simulink model "RefModel_SimpleUavMotion"  (R2020a)
settings: Solver=ode1  StartTime=0.0  StopTime=10.0  FixedStep=Ts_Task.Ts_base  RelTol=1e-3
undefined symbols (not defined in the file or in its folder): alt, DiscIntNeverNeededParam, ENUM_FlightControlMode, ENUM_UAVMode, eulerd_yaw_pitch_roll, initialAlignmentCompleteFlag, isHeadingRotateFlag, isNavFilterGood, latd, lla, lond, pitchd, posNED, refloc, rolld, TASK_SET, Ts_SimpleUavMotion, velNED, yawd
libraries: simulink x16, discretizedSecondOrderIntegrator x3, discretizing x2
(part 1 of 2)
settings Model: Creator=sl  LastModifiedBy=Administrator
settings DataIOCC: SaveOutput=off  SaveTime=off
settings OptimizationCC: DefaultParameterBehavior=Inlined  EnhancedBackFolding=on  PassReuseOutputArgsAs=Individual arguments  ZeroExternalMemoryAtStartup=off  ZeroInternalMemoryAtStartup=off  OptimizeBlockOrder=speed  DifferentSizesBufferReuse=on  EfficientTunableParamExpr=on
settings DebuggingCC: InheritedTsInSrcMsg=none  ParameterPrecisionLossMsg=none  ParameterTunabilityLossMsg=error  UnconnectedInputMsg=none  UnconnectedOutputMsg=none  UnconnectedLineMsg=none  SFUnusedDataAndEventsDiag=none
settings HardwareCC: ProdBitPerPointer=32  ProdBitPerSizeT=32  ProdBitPerPtrDiffT=32  ProdLargestAtomicInteger=Long  ProdLargestAtomicFloat=Double  ProdWordSize=32  ProdHWDeviceType=ARM Compatible->ARM Cortex
settings ModelReferenceCC: ModelReferenceNumInstancesAllowed=Single
settings SFSimCC: MATLABDynamicMemAlloc=off
settings RTWCC: SystemTargetFile=ert.tlc  TemplateMakefile=ert_default_tmf  GenerateReport=on  IncludeHyperlinkInReport=on  LaunchReport=on  GenerateTraceInfo=on  GenerateTraceReport=on  GenerateTraceReportSl=on  GenerateTraceReportSf=on  GenerateTraceReportEml=on
settings CodeAppCC: ForceParamTrailComments=on  IgnoreCustomStorageClasses=off  MaxIdLength=48  OperatorAnnotations=on  SimulinkDataObjDesc=on  SFDataObjDesc=on  InsertBlockDesc=on
settings ERTTargetCC: TargetLangStandard=C99 (ISO)  GenerateSampleERTMain=on  CombineOutputUpdateFcns=off  LogVarNameModifier=none  SupportVariableSizeSignals=on  InlinedParameterPlacement=NonHierarchical  ERTCustomFileTemplate=example_file_process.tlc

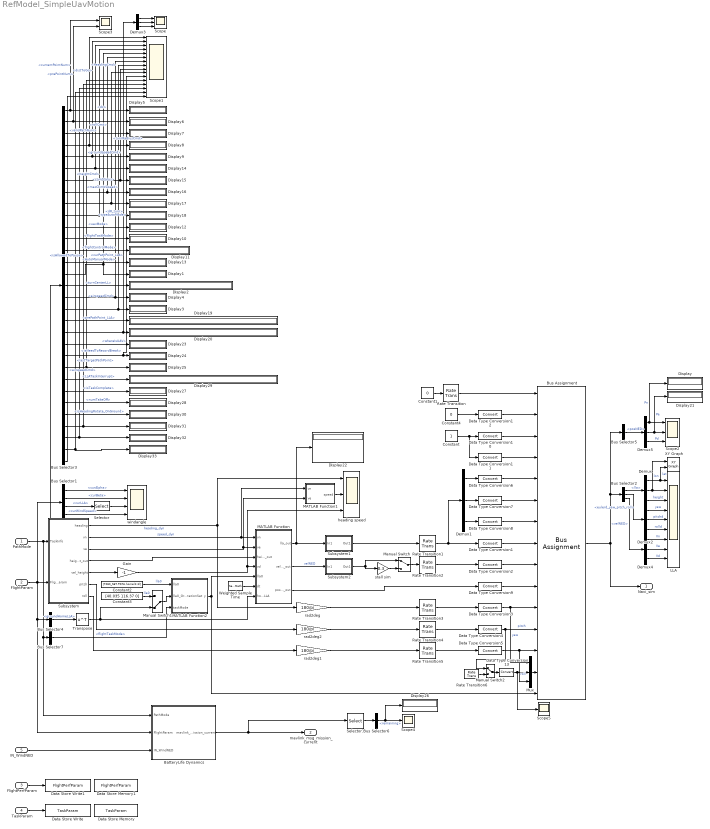
== system RefModel_SimpleUavMotion ==
  PathMode : Inport  OutDataTypeStr=Bus: BUS_TASK_PATH_OutParam
  FlightParam : Inport  Port=2  OutDataTypeStr=Bus: BUS_TASK_COMMON_OutParam
  FlightPerfParam : Inport  Port=3  OutDataTypeStr=Bus: BUS_FLIGHTPERF_PARAM  BusOutputAsStruct=on
  TaskParam : Inport  Port=4  OutDataTypeStr=Bus: BUS_TASK_PATH_AlgoParam  BusOutputAsStruct=on
  IN_WindNED : Inport  Port=5  OutDataTypeStr=Bus: BUS_NAVI_GlobalWindEst
  BatteryLife Dynamics : Subsystem
  Bus Assignment : BusAssignment  AssignedSignals=isHeadingRotateFlag,initialAlignmentCompleteFlag,isNavFilterGood,latd,lond,alt,lla,velNED,posNED,yawd,pitchd,rolld,eulerd_yaw_pitch_roll,refloc
  Bus Selector1 : BusSelector  OutputSignals=curAlpha,curBeta,curLLA,curWindSpeed
  Bus Selector2 : BusSelector  OutputSignals=lla,eulerd_yaw_pitch_roll,velNED
  Bus Selector3 : BusSelector  OutputSignals=currentPointNum,prePointNum,validPathNum,headingCmd,distToGo,dz,groundspeedCmd,rollCmd,turnRadiusCmd,heightCmd,uavMode,flightTaskMode,flightControlMode,AutoManualMode,dR_turn,turnCenterLL,comStatus,maxClimbSpeed,prePathPoint_LLA,curPathPoint_LLA,whereIsUAV,typeAutoMode,airspeedCmd,LLATaskInterrupt,isTaskComplete,numTakeOff,isHeadingRotate_OnGround,isAllowedToPause,isNeedToRecordBreak,lastTargetPathPoint,airspeedCmd
  Bus Selector4 : BusSelector  OutputSignals=groundHomeLLA
  Bus Selector5 : BusSelector  OutputSignals=posNED
  Bus Selector6 : BusSelector  OutputSignals=remaining
  Bus Selector7 : BusSelector  OutputSignals=flightTaskMode
  Constant : Constant
  Constant1 : Constant  Value=0  OutDataTypeStr=Bus: BUS_NAVI_TO_FIRM
  Constant2 : Constant  Value=[TASK_SET.PATH.home(1:3)]
  Constant3 : Constant  Value=[40.035 116.37 0]
  Constant4 : Constant  Value=0
  Data Store Memory : DataStoreMemory  DataStoreName=TaskParam  ReadBeforeWriteMsg=warning  WriteAfterWriteMsg=warning  WriteAfterReadMsg=warning  ShowAdditionalParam=off  OutDataTypeStr=Bus: BUS_TASK_PATH_AlgoParam  Dimensions=1
  Data Store Memory1 : DataStoreMemory  DataStoreName=FlightPerfParam  ReadBeforeWriteMsg=warning  WriteAfterWriteMsg=warning  WriteAfterReadMsg=warning  ShowAdditionalParam=off  OutDataTypeStr=Bus: BUS_FLIGHTPERF_PARAM  Dimensions=1
  Data Store Write : DataStoreWrite  DataStoreName=TaskParam
  Data Store Write1 : DataStoreWrite  DataStoreName=FlightPerfParam
  Data Type Conversion{1..13} (13 alike) : DataTypeConversion
  Demux{,1..5} (6 alike) : Demux  Outputs=3
  Display{,1..33} (34 alike) : Display
  Gain : Gain  Gain=-1
  LLA : Scope  NumInputPorts=9
  MATLAB Function : MATLAB Function  TreatAsAtomicUnit=on
  MATLAB Function1 : MATLAB Function  TreatAsAtomicUnit=on
  MATLAB Function2 : MATLAB Function  TreatAsAtomicUnit=on
  Manual Switch : ManualSwitch
  Manual Switch1 : ManualSwitch  CurrentSetting=0
  Manual Switch2 : ManualSwitch
  Mux : Mux  Inputs=3
  Rate Transition{,1..6} (7 alike) : RateTransition
  Scope : Scope  NumInputPorts=3
  Scope1 : Scope  NumInputPorts=16
  Scope2 : Scope  NumInputPorts=3
  Scope3 : Scope  NumInputPorts=2
  Scope4 : Scope
  Scope5 : Scope
  Selector : Selector  InputPortWidth=3  IndexOptions=Index vector (dialog)  Indices=3  OutputSizes=1
  Selector1 : Selector  InputPortWidth=3  IndexOptions=Index vector (dialog)  Indices=1  OutputSizes=1
  Subsystem : Subsystem
  Subsystem1 : Subsystem
  Subsystem2 : Subsystem
  Transpose : Math  Operator=transpose  SaturateOnIntegerOverflow=on
  Weighted Sample Time : SampleTimeMath  TsampMathOp=Ts Only
  XY Graph : simulink/Sinks/XY Graph  xmin=116.34  xmax=116.42  ymin=40.02  ymax=40.08  st=-1
  heading speed : Scope  NumInputPorts=3
  rad2deg : Gain  Gain=180/pi
  rad2deg1 : Gain  Gain=180/pi
  rad2deg2 : Gain  Gain=180/pi
  stall sim : Gain  Gain=0.3
  windangle : Scope  NumInputPorts=4
  Navi_sim : Outport  OutDataTypeStr=Bus: BUS_NAVI_TO_FIRM
  mavlink_msg_mission_current : Outport  Port=2  OutDataTypeStr=Bus: mavlink_msg_mission_current  BusOutputAsStruct=on
  wires:
  Data Type Conversion2/1 -> Bus Assignment/9
  Bus Selector3/16 -> Display2/1  "<turnCenterLL>"
  Rate Transition5/1 -> Data Type Conversion5/1
  Data Type Conversion5/1 -> Mux/3, Bus Assignment/13  "roll"
  Bus Selector3/15 -> Display1/1, Scope1/5  "<dR_turn>"
  Weighted Sample Time/1 -> MATLAB Function/6(dt)
  Data Type Conversion4/1 -> Manual Switch2/1, Bus Assignment/12  "pitch"
  Data Type Conversion1/1 -> Bus Assignment/8
  Rate Transition4/1 -> Data Type Conversion4/1
  Bus Selector3/14 -> Display13/1  "<AutoManualMode>"
  Subsystem/4(height_out) -> MATLAB Function/3(height_out)
  Data Type Conversion7/1 -> Bus Assignment/6
  Data Type Conversion6/1 -> Bus Assignment/5
  Subsystem/6(pitch) -> rad2deg2/1
  Demux1/3 -> Data Type Conversion8/1
  Rate Transition1/1 -> Demux1/1, Data Type Conversion1/1
  Data Type Conversion8/1 -> Bus Assignment/7
  Demux1/2 -> Data Type Conversion7/1
  Demux1/1 -> Data Type Conversion6/1
  Bus Selector3/13 -> Display11/1  "<flightControlMode>"
  Bus Selector3/6 -> Scope1/3, Display14/1  "<dz>"
  rad2deg1/1 -> Rate Transition5/1
  Rate Transition/1 -> Bus Assignment/1
  PathMode/1 -> Bus Selector7/1, BatteryLife Dynamics/1(PathMode), Bus Selector3/1, Subsystem/1(TaskInfo)
  Bus Selector3/2 -> Scope3/2, Display6/1  "<prePointNum>"
  Bus Selector3/8 -> Scope1/6, Display16/1  "<rollCmd>"
  Bus Selector3/10 -> Scope1/4, Display18/1  "<heightCmd>"
  Bus Selector3/1 -> Scope3/1, Display5/1  "<currentPointNum>"
  Bus Selector3/7 -> Scope1/9, Display15/1  "<groundspeedCmd>"
  Bus Selector3/5 -> Scope1/2, Display9/1  "<distToGo>"
  Constant2/1 -> MATLAB Function2/1(lla0)  "lla0"
  Bus Selector3/4 -> Scope1/1, Display8/1  "<headingCmd>"
  rad2deg/1 -> Rate Transition3/1
  Bus Selector3/11 -> Display12/1  "<uavMode>"
  Subsystem/2(vn) -> MATLAB Function1/1(vn), MATLAB Function/1(vn)  "speed_dyn"
  Subsystem/1(heading) -> heading speed/1, rad2deg/1  "heading_dyn"
  Bus Selector3/9 -> Scope1/10, Display17/1  "<turnRadiusCmd>"
  Rate Transition2/1 -> Data Type Conversion2/1
  Bus Selector3/3 -> Display7/1  "<validPathNum>"
  Bus Selector3/12 -> Display10/1  "<flightTaskMode>"
  Subsystem/5(vel_height) -> Gain/1
  Constant1/1 -> Rate Transition/1
  Subsystem/7(roll) -> rad2deg1/1
  Data Type Conversion3/1 -> Mux/1, Bus Assignment/11  "yaw"
  Mux/1 -> Bus Assignment/14
  FlightParam/1 -> BatteryLife Dynamics/2(FlightParam), Bus Selector4/1, Bus Selector1/1, Subsystem/2(FlightParam)
  rad2deg2/1 -> Rate Transition4/1
  Subsystem/3(ve) -> MATLAB Function1/2(ve), MATLAB Function/2(ve)
  MATLAB Function1/1(speed) -> heading speed/2
  MATLAB Function/2(velNED_out) -> Subsystem2/1(In1)  "velNED"
  Manual Switch/1 -> Rate Transition2/1
  stall sim/1 -> Manual Switch/2
  Demux2/2 -> LLA/5  "pitchd"
  Demux2/3 -> LLA/6  "rolld"
  Demux/1 -> XY Graph/2, LLA/1  "lat"
  Bus Assignment/1 -> Bus Selector2/1, Bus Selector5/1, Navi_sim/1
  Demux/3 -> LLA/3  "height"
  Demux2/1 -> LLA/4  "yaw"
  Demux/2 -> XY Graph/1, LLA/2  "lon"
  Bus Selector2/2 -> Demux2/1  "<eulerd_yaw_pitch_roll>"
  Bus Selector2/1 -> Demux/1  "<lla>"
  Bus Selector3/17 -> Scope1/7, Display4/1  "<comStatus>"
  Bus Selector3/18 -> Scope1/8, Display3/1  "<maxClimbSpeed>"
  Bus Selector3/20 -> Demux3/1, Display20/1  "<curPathPoint_LLA>"
  Rate Transition3/1 -> Data Type Conversion3/1
  Demux3/1 -> Scope/1
  Demux3/2 -> Scope/2
  Demux3/3 -> Scope/3
  MATLAB Function/1(lla_out) -> Display22/1, Subsystem1/1(In1)
  Subsystem1/1(Out1) -> Rate Transition1/1
  Subsystem2/1(Out1) -> Manual Switch/1, stall sim/1
  FlightPerfParam/1 -> Data Store Write1/1
  MATLAB Function2/1(y) -> MATLAB Function/5(lla0), Bus Assignment/15
  Manual Switch1/1 -> MATLAB Function2/2(lla0_GroundStationSet)
  Bus Selector4/1 -> Transpose/1  "<groundHomeLLA>"
  Constant3/1 -> Manual Switch1/1  "lla0"
  Bus Selector1/1 -> windangle/1  "<curAlpha>"
  Bus Selector1/2 -> windangle/2  "<curBeta>"
  Bus Selector2/3 -> Demux4/1  "<velNED>"
  Demux4/1 -> LLA/7  "Vn"
  Demux4/2 -> LLA/8  "Ve"
  Demux4/3 -> LLA/9  "Vd"
  Transpose/1 -> Manual Switch1/2, MATLAB Function/7(homeLLA)
  Bus Selector1/3 -> Selector/1  "<curLLA>"
  Selector/1 -> windangle/3
  Bus Selector1/4 -> windangle/4  "<curWindSpeed>"
  Gain/1 -> heading speed/3, MATLAB Function/4(vd)
  Data Type Conversion9/1 -> Bus Assignment/10
  Demux5/1 -> Display/1, Scope2/1  "Pn"
  Demux5/2 -> Display21/1, Scope2/2  "Pe"
  Demux5/3 -> Scope2/3  "Pd"
  Bus Selector5/1 -> Demux5/1  "<posNED>"
  MATLAB Function/3(posNED_out) -> Data Type Conversion9/1
  Constant/1 -> Data Type Conversion11/1, Data Type Conversion10/1
  Data Type Conversion10/1 -> Bus Assignment/3
  Bus Selector3/19 -> Display19/1  "<prePathPoint_LLA>"
  Bus Selector3/21 -> Display23/1  "<whereIsUAV>"
  Bus Selector3/22 -> Scope1/11, Display24/1  "<typeAutoMode>"
  Bus Selector3/23 -> Display25/1, Scope1/12  "<airspeedCmd>"
  Data Type Conversion11/1 -> Bus Assignment/4
  BatteryLife Dynamics/1(mavlink_msg_mission_current) -> Selector1/1, mavlink_msg_mission_current/1
  Selector1/1 -> Bus Selector6/1
  Bus Selector6/1 -> Display26/1, Scope4/1  "<remaining>"
  Bus Selector7/1 -> MATLAB Function2/3(taskMode)  "<flightTaskMode>"
  Bus Selector3/24 -> Display29/1  "<LLATaskInterrupt>"
  Bus Selector3/25 -> Display27/1  "<isTaskComplete>"
  Bus Selector3/26 -> Display28/1  "<numTakeOff>"
  Constant4/1 -> Data Type Conversion12/1
  Data Type Conversion12/1 -> Bus Assignment/2
  Bus Selector3/27 -> Display30/1  "<isHeadingRotate_OnGround>"
  IN_WindNED/1 -> BatteryLife Dynamics/3(IN_WindNED)
  Bus Selector3/28 -> Scope1/13, Display31/1  "<isAllowedToPause>"
  Bus Selector3/29 -> Scope1/14, Display32/1  "<isNeedToRecordBreak>"
  Bus Selector3/30 -> Display33/1, Scope1/15  "<lastTargetPathPoint>"
  Bus Selector3/31 -> Scope1/16  "<airspeedCmd>"
  TaskParam/1 -> Data Store Write/1
  ? -> Rate Transition6/1
  Manual Switch2/1 -> Data Type Conversion13/1
  Data Type Conversion13/1 -> Scope5/1, Mux/2
  Rate Transition6/1 -> Manual Switch2/2

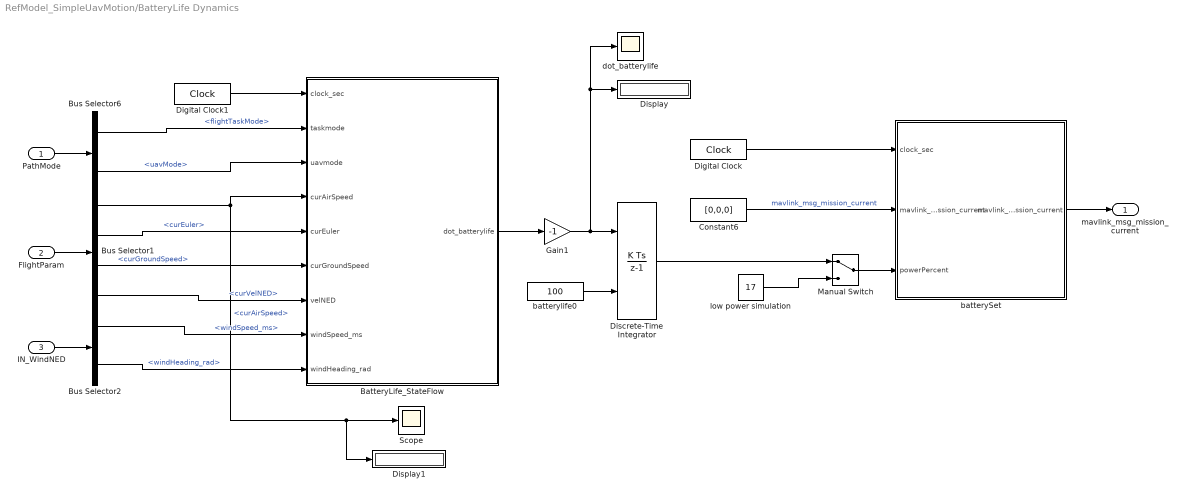
== system RefModel_SimpleUavMotion/BatteryLife Dynamics ==
  PathMode : Inport
  FlightParam : Inport  Port=2
  IN_WindNED : Inport  Port=3
  BatteryLife_StateFlow : Stateflow chart  TreatAsAtomicUnit=on
  Bus Selector1 : BusSelector  OutputSignals=curAirSpeed,curEuler,curGroundSpeed,curVelNED
  Bus Selector2 : BusSelector  OutputSignals=windSpeed_ms,windHeading_rad
  Bus Selector6 : BusSelector  OutputSignals=flightTaskMode,uavMode
  Constant6 : Constant  Value=[0,0,0]  OutDataTypeStr=Bus: mavlink_msg_mission_current
  Digital Clock : DigitalClock  SampleTime=-1
  Digital Clock1 : DigitalClock  SampleTime=-1
  Discrete-Time Integrator : DiscreteIntegrator  InitialConditionSource=external  SampleTime=-1  ICPrevOutput=DiscIntNeverNeededParam  ICPrevScaledInput=DiscIntNeverNeededParam
  Display : Display
  Display1 : Display
  Gain1 : Gain  Gain=-1
  Manual Switch : ManualSwitch
  Scope : Scope
  batterySet : MATLAB Function  TreatAsAtomicUnit=on
  batterylife0 : Constant  Value=100
  dot_batterylife : Scope
  low power simulation : Constant  Value=17
  mavlink_msg_mission_current : Outport  OutDataTypeStr=Bus: mavlink_msg_mission_current  BusOutputAsStruct=on
  wires:
  batterylife0/1 -> Discrete-Time Integrator/2
  Gain1/1 -> dot_batterylife/1, Display/1, Discrete-Time Integrator/1
  Digital Clock1/1 -> BatteryLife_StateFlow/1(clock_sec)
  BatteryLife_StateFlow/1(dot_batterylife) -> Gain1/1
  Bus Selector6/1 -> BatteryLife_StateFlow/2(taskmode)  "<flightTaskMode>"
  Constant6/1 -> batterySet/2("mavlink_msg_mission_current ")  "mavlink_msg_mission_current"
  batterySet/1(mavlink_msg_mission_current) -> mavlink_msg_mission_current/1
  Digital Clock/1 -> batterySet/1(clock_sec)
  Bus Selector6/2 -> BatteryLife_StateFlow/3(uavmode)  "<uavMode>"
  PathMode/1 -> Bus Selector6/1
  FlightParam/1 -> Bus Selector1/1
  Bus Selector1/1 -> Display1/1, Scope/1, BatteryLife_StateFlow/4(curAirSpeed)  "<curAirSpeed>"
  Bus Selector1/2 -> BatteryLife_StateFlow/5(curEuler)  "<curEuler>"
  IN_WindNED/1 -> Bus Selector2/1
  Bus Selector2/1 -> BatteryLife_StateFlow/8(windSpeed_ms)  "<windSpeed_ms>"
  Bus Selector2/2 -> BatteryLife_StateFlow/9(windHeading_rad)  "<windHeading_rad>"
  Bus Selector1/3 -> BatteryLife_StateFlow/6(curGroundSpeed)  "<curGroundSpeed>"
  Discrete-Time Integrator/1 -> Manual Switch/1
  low power simulation/1 -> Manual Switch/2
  Manual Switch/1 -> batterySet/3(powerPercent)
  Bus Selector1/4 -> BatteryLife_StateFlow/7(velNED)  "<curVelNED>"

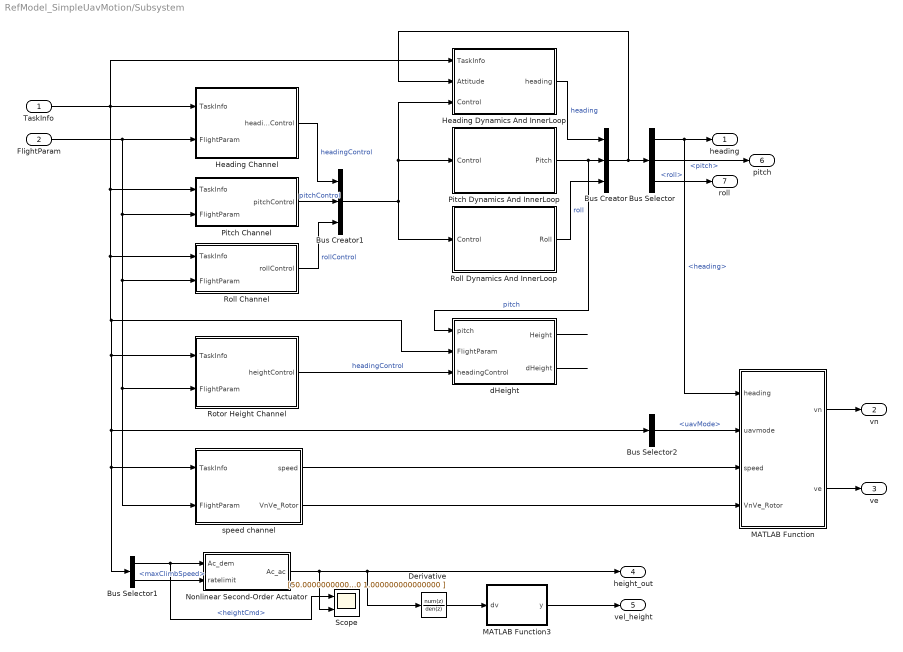
== system RefModel_SimpleUavMotion/Subsystem ==
  TaskInfo : Inport
  FlightParam : Inport  Port=2
  Bus Creator : BusCreator  Inputs=3
  Bus Creator1 : BusCreator  Inputs=3
  Bus Selector : BusSelector  OutputSignals=heading,pitch,roll
  Bus Selector1 : BusSelector  OutputSignals=heightCmd,maxClimbSpeed
  Bus Selector2 : BusSelector  OutputSignals=uavMode
  Derivative : DiscreteTransferFcn  Numerator=[50.000000000000000 -50.000000000000000 ]  Denominator=[1.000000000000000 1.000000000000000 ]  SampleTime=Ts_SimpleUavMotion.Ts_base
  Heading Channel : Subsystem
  Heading Dynamics And InnerLoop : Subsystem
  MATLAB Function : MATLAB Function  TreatAsAtomicUnit=on
  MATLAB Function3 : MATLAB Function  TreatAsAtomicUnit=on
  Nonlinear Second-Order Actuator : Subsystem  AncestorBlock=aerolibactuator/Nonlinear Second-Order Actuator  mask(NonlinearSecondOrderActuator){wn_fin=1, z_fin=0.7, fin_max=1e4, fin_min=0, fin_maxrate=5, fin_act_0=0, fin_act_vel=0}
      mask prompts: wn_fin "aeroblks:aeroblkactuator:blockNonlinearSecondOrderActuatorParamNaturalfrequency"; z_fin "aeroblks:aeroblkactuator:blockNonlinearSecondOrderActuatorParamDampingratio"; fin_max "aeroblks:aeroblkactuator:blockNonlinearSecondOrderActuatorParamMaximumdeflection"; fin_min "aeroblks:aeroblkactuator:blockNonlinearSecondOrderActuatorParamMinimumdeflection"; fin_maxrate "aeroblks:aeroblkactuator:blockNonlinearSecondOrderActuatorParamRatelimit"; fin_act_0 "aeroblks:aeroblkactuator:blockNonlinearSecondOrderActuatorParamInitialposition"; fin_act_vel "aeroblks:aeroblkactuator:blockNonlinearSecondOrderActuatorParamInitialvelocity"
      mask help: aeroblks:aeroblkactuator:blockNonlinearSecondOrderActuatorDesc
      mask init:
      | par = [fin_max fin_min fin_act_0 fin_act_vel fin_maxrate];
      | aeroicon('aeroblkactuator',par)
      mask Help: eval('asbhelp');
      mask DialogControl wn_fin Prompt: Natural frequency:
      mask DialogControl z_fin Prompt: Damping ratio:
      mask DialogControl fin_max Prompt: Maximum deflection:
      mask DialogControl fin_min Prompt: Minimum deflection:
      mask DialogControl fin_maxrate Prompt: Rate limit:
      mask DialogControl fin_act_0 Prompt: Initial position:
      mask DialogControl fin_act_vel Prompt: Initial velocity:
      mask Display:
      | port_label('input',1,'A_{demand}','texmode','on');
      | port_label('output',1,'A_{actual}','texmode','on');
  Pitch Channel : Subsystem
  Pitch Dynamics And InnerLoop : Subsystem
  Roll Channel : Subsystem
  Roll Dynamics And InnerLoop : Subsystem
  Rotor Height Channel : Subsystem
  Scope : Scope  NumInputPorts=2
  dHeight : Subsystem
  speed channel : Subsystem
  heading : Outport
  vn : Outport  Port=2
  ve : Outport  Port=3
  height_out : Outport  Port=4
  vel_height : Outport  Port=5
  pitch : Outport  Port=6
  roll : Outport  Port=7
  wires:
  speed channel/1(speed) -> MATLAB Function/3(speed)
  Derivative/1 -> MATLAB Function3/1(dv)
  MATLAB Function3/1(y) -> vel_height/1
  Heading Dynamics And InnerLoop/1(heading) -> Bus Creator/1  "heading"
  Bus Creator/1 -> Bus Selector/1, Heading Dynamics And InnerLoop/2(Attitude)
  Bus Selector/3 -> roll/1  "<roll>"
  Bus Selector/1 -> MATLAB Function/1(heading), heading/1  "<heading>"
  Roll Channel/1(rollControl) -> Bus Creator1/3  "rollControl"
  Heading Channel/1(headingControl) -> Bus Creator1/1  "headingControl"
  Pitch Channel/1(pitchControl) -> Bus Creator1/2  "pitchControl"
  Bus Creator1/1 -> Roll Dynamics And InnerLoop/1(Control), Pitch Dynamics And InnerLoop/1(Control), Heading Dynamics And InnerLoop/3(Control)
  Pitch Dynamics And InnerLoop/1(Pitch) -> dHeight/1(pitch), Bus Creator/2  "pitch"
  Roll Dynamics And InnerLoop/1(Roll) -> Bus Creator/3  "roll"
  TaskInfo/1 -> Roll Channel/1(TaskInfo), dHeight/2(FlightParam), Bus Selector1/1, speed channel/1(TaskInfo), Bus Selector2/1, Rotor Height Channel/1(TaskInfo), Pitch Channel/1(TaskInfo), Heading Dynamics And InnerLoop/1(TaskInfo), Heading Channel/1(TaskInfo)
  Bus Selector1/1 -> Scope/1, Nonlinear Second-Order Actuator/1(Ac_dem)  "<heightCmd>"
  FlightParam/1 -> speed channel/2(FlightParam), Rotor Height Channel/2(FlightParam), Roll Channel/2(FlightParam), Pitch Channel/2(FlightParam), Heading Channel/2(FlightParam)
  Bus Selector/2 -> pitch/1  "<pitch>"
  Rotor Height Channel/1(heightControl) -> dHeight/3(headingControl)  "headingControl"
  dHeight/1(Height) -> ?
  dHeight/2(dHeight) -> ?
  Bus Selector2/1 -> MATLAB Function/2(uavmode)  "<uavMode>"
  speed channel/2(VnVe_Rotor) -> MATLAB Function/4(VnVe_Rotor)
  MATLAB Function/1(vn) -> vn/1
  MATLAB Function/2(ve) -> ve/1
  Bus Selector1/2 -> Nonlinear Second-Order Actuator/2(ratelimit)  "<maxClimbSpeed>"
  Nonlinear Second-Order Actuator/1(Ac_ac) -> Scope/2, Derivative/1, height_out/1

== system RefModel_SimpleUavMotion/Subsystem1 ==
  In1 : Inport
  Add : Sum
  Random Number : RandomNumber  Seed=[23,123,15]
  g : Gain  Gain=[0.05/111e3,0.05/111e3,0.1]
  Out1 : Outport
  wires:
  Random Number/1 -> g/1
  g/1 -> Add/1
  In1/1 -> Add/2
  Add/1 -> Out1/1

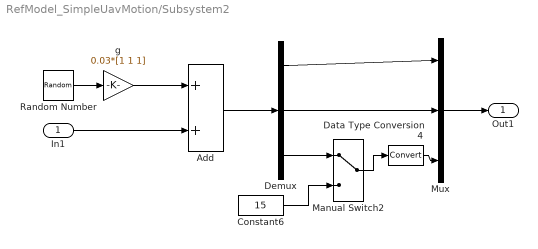
== system RefModel_SimpleUavMotion/Subsystem2 ==
  In1 : Inport
  Add : Sum
  Constant6 : Constant  Value=15
  Data Type Conversion4 : DataTypeConversion
  Demux : Demux  Outputs=3
  Manual Switch2 : ManualSwitch
  Mux : Mux  Inputs=3
  Random Number : RandomNumber  Seed=[652,231,255]
  g : Gain  Gain=0.03*[1 1 1]
  Out1 : Outport
  wires:
  In1/1 -> Add/2
  g/1 -> Add/1
  Random Number/1 -> g/1
  Demux/1 -> Mux/1
  Demux/2 -> Mux/2
  Mux/1 -> Out1/1
  Add/1 -> Demux/1
  Demux/3 -> Manual Switch2/1
  Manual Switch2/1 -> Data Type Conversion4/1
  Data Type Conversion4/1 -> Mux/3
  Constant6/1 -> Manual Switch2/2

== system RefModel_SimpleUavMotion/Subsystem/Heading Channel ==
  TaskInfo : Inport
  FlightParam : Inport  Port=2
  Bus Selector1 : BusSelector  OutputSignals=curEuler
  Bus Selector3 : BusSelector  OutputSignals=headingCmd,uavMode
  Heading Controller : Subsystem
  Selector : Selector  InputPortWidth=3  IndexOptions=Index vector (dialog)  Indices=1  OutputSizes=1
  headingControl : Outport
  wires:
  TaskInfo/1 -> Bus Selector3/1
  Heading Controller/1(headingControl) -> headingControl/1
  Bus Selector3/2 -> Heading Controller/2(uavMode)  "<uavMode>"
  Bus Selector3/1 -> Heading Controller/1(headingCmd)  "<headingCmd>"
  FlightParam/1 -> Bus Selector1/1
  Selector/1 -> Heading Controller/3(heading)
  Bus Selector1/1 -> Selector/1  "<curEuler>"

== system RefModel_SimpleUavMotion/Subsystem/Heading Dynamics And InnerLoop ==
  TaskInfo : Inport
  Attitude : Inport  Port=2
  Control : Inport  Port=3
  Bus Selector1 : BusSelector  OutputSignals=roll
  Bus Selector2 : BusSelector  OutputSignals=headingControl
  Bus Selector3 : BusSelector  OutputSignals=groundspeedCmd
  HeadingMotion : Subsystem
  heading : Outport
  wires:
  TaskInfo/1 -> Bus Selector3/1
  Bus Selector3/1 -> HeadingMotion/3(speed)  "<groundspeedCmd>"
  HeadingMotion/1(heading) -> heading/1  "heading"
  Attitude/1 -> Bus Selector1/1
  Control/1 -> Bus Selector2/1
  Bus Selector1/1 -> HeadingMotion/1(roll)  "<roll>"
  Bus Selector2/1 -> HeadingMotion/2(headingControl)  "<headingControl>"

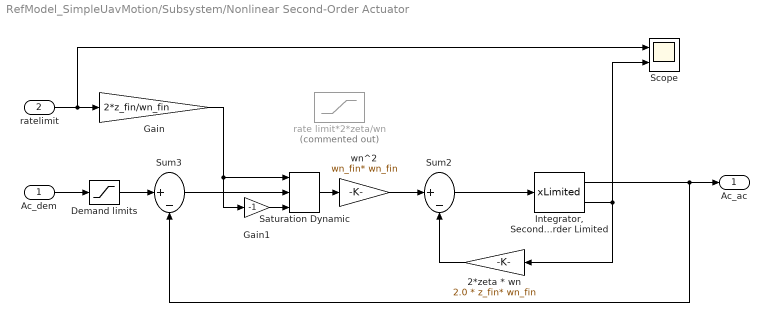
== system RefModel_SimpleUavMotion/Subsystem/Nonlinear Second-Order Actuator ==
  Ac_dem : Inport
  ratelimit : Inport  Port=2
  2*zeta * wn : Gain  Gain=2.0 * z_fin* wn_fin  SaturateOnIntegerOverflow=on  OutDataTypeStr=Inherit: Same as input  ParamDataTypeStr=Inherit: Same as input
  Demand limits : Saturate  UpperLimit=fin_max  LowerLimit=fin_min
  Gain : Gain  Gain=2*z_fin/wn_fin
  Gain1 : Gain  Gain=-1
  "Integrator, Second-Order Limited" : discretizedSecondOrderIntegrator/xLimited  ICSourceX=internal  ICX=fin_act_0  LimitX=on  UpperLimitX=fin_max  LowerLimitX=fin_min  ICSourceDXDT=internal  ICDXDT=fin_act_vel  LimitDXDT=on  UpperLimitDXDT=fin_maxrate  LowerLimitDXDT=-fin_maxrate  ExternalReset=none  IgnoreStateLimitsAndResetForLinearization=off  ReinitDXDTwhenXreachesSaturation=off  ShowOutput=both  GainValue=1.0  SampleTime=Ts_SimpleUavMotion.Ts_base  IntegratorMethod=Integration: Forward Euler
      settings: SourceProductBaseCode=SL
  Saturation Dynamic : simulink/Discontinuities/Saturation Dynamic  OutMin=[]  OutMax=[]  OutDataTypeStr=Inherit: Same as second input  OutDataType=fixdt(1, 16)  OutScaling=2^-10  DoSatur=off
  Scope : Scope  NumInputPorts=2
  Sum2 : Sum  Inputs=|+-  InputSameDT=on  SaturateOnIntegerOverflow=on  OutDataTypeStr=Inherit: Same as first input
  Sum3 : Sum  Inputs=|+-  InputSameDT=on  SaturateOnIntegerOverflow=on  OutDataTypeStr=Inherit: Same as first input
  rate limit*2*zeta/wn : Saturate  Commented=on  UpperLimit=fin_maxrate*2*z_fin/wn_fin  LowerLimit=-fin_maxrate*2*z_fin/wn_fin
  wn^2 : Gain  Gain=wn_fin* wn_fin  SaturateOnIntegerOverflow=on  OutDataTypeStr=Inherit: Same as input  ParamDataTypeStr=Inherit: Same as input
  Ac_ac : Outport  InitialOutput=0  VectorParamsAs1DForOutWhenUnconnected=off
  wires:
  Ac_dem/1 -> Demand limits/1
  Demand limits/1 -> Sum3/1
  Saturation Dynamic/1 -> wn^2/1
  Sum3/1 -> Saturation Dynamic/2
  2*zeta * wn/1 -> Sum2/2
  Sum2/1 -> "Integrator, Second-Order Limited"/1
  wn^2/1 -> Sum2/1
  "Integrator, Second-Order Limited"/1 -> Sum3/2, Ac_ac/1
  "Integrator, Second-Order Limited"/2 -> Scope/2, 2*zeta * wn/1
  Gain/1 -> Gain1/1, Saturation Dynamic/1
  Gain1/1 -> Saturation Dynamic/3
  ratelimit/1 -> Scope/1, Gain/1

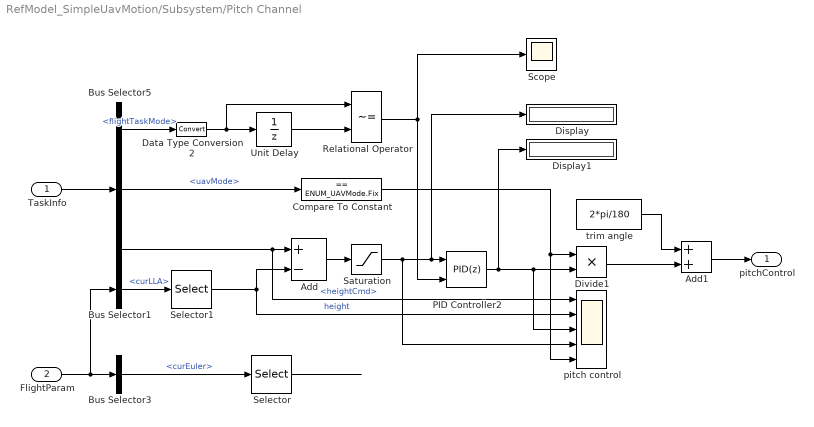
== system RefModel_SimpleUavMotion/Subsystem/Pitch Channel ==
  TaskInfo : Inport
  FlightParam : Inport  Port=2
  Add : Sum  Inputs=+-
  Add1 : Sum
  Bus Selector1 : BusSelector  OutputSignals=curLLA
  Bus Selector3 : BusSelector  OutputSignals=curEuler
  Bus Selector5 : BusSelector  OutputSignals=flightTaskMode,uavMode,heightCmd
  Compare To Constant : simulink/Logic and Bit Operations/Compare To Constant  relop===  const=ENUM_UAVMode.Fix  OutDataTypeStr=boolean
  Data Type Conversion2 : DataTypeConversion
  Display : Display
  Display1 : Display
  Divide1 : Product  Inputs=**
  PID Controller2 : simulink/Continuous/PID Controller  Controller=PID  Form=Parallel  TimeDomain=Discrete-time  UseExternalTs=off  SampleTime=Ts_SimpleUavMotion.Ts_base  IntegratorMethod=Forward Euler  FilterMethod=Forward Euler  ControllerParametersSource=internal  P=0.04  I=0  D=0  UseFilter=off  N=24.542109027781645  TunerSelectOption=Transfer Function Based (PID Tuner App)  InitialConditionSource=internal  InitialConditionForIntegrator=0  InitialConditionForFilter=0  DifferentiatorICPrevScaledInput=0  ExternalReset=rising  TrackingMode=off  Kt=1  LimitOutput=on  UpperSaturationLimit=30*pi/180  LowerSaturationLimit=-30*pi/180  LinearizeAsGain=on  AntiWindupMode=back-calculation  Kb=1  POutMin=[]  POutMax=[]  IOutMin=[]  IOutMax=[]  DOutMin=[]  DOutMax=[]  NOutMin=[]  NOutMax=[]  SumOutMin=[]  SumOutMax=[]  SaturationOutMin=[]  SaturationOutMax=[]  PParamMin=[]  PParamMax=[]  IParamMin=[]  IParamMax=[]  DParamMin=[]  DParamMax=[]  NParamMin=[]  NParamMax=[]  KbParamMin=[]  KbParamMax=[]  KtParamMin=[]  KtParamMax=[]  KbOutMin=[]  KbOutMax=[]  KtOutMin=[]  KtOutMax=[]  IntegratorOutMin=[]  IntegratorOutMax=[]  FilterOutMin=[]  FilterOutMax=[]  SumI1OutMin=[]  SumI1OutMax=[]  SumI2OutMin=[]  SumI2OutMax=[]  SumI3OutMin=[]  SumI3OutMax=[]  SumI4OutMin=[]  SumI4OutMax=[]  SumDOutMin=[]  SumDOutMax=[]  DifferentiatorOutMin=[]  DifferentiatorOutMax=[]  FilterDiffOutCoefMin=[]  FilterDiffOutCoefMax=[]  ReciprocalOutMin=[]  ReciprocalOutMax=[]  SumDenOutMin=[]  SumDenOutMax=[]  SumNumOutMin=[]  SumNumOutMax=[]  DivideOutMin=[]  DivideOutMax=[]  UdiffTsProdOutMin=[]  UdiffTsProdOutMax=[]  NTsProdOutMin=[]  NTsProdOutMax=[]  UintegralTsProdOutMin=[]  UintegralTsProdOutMax=[]  UngainTsProdOutMin=[]  UngainTsProdOutMax=[]  IntegratorContinuousStateAttributes=''  IntegratorStateMustResolveToSignalObject=off  IntegratorRTWStateStorageClass=Auto  FilterContinuousStateAttributes=''  FilterStateMustResolveToSignalObject=off  FilterRTWStateStorageClass=Auto  ParallelPVariant=InternalParameters  IdealPVariant=Disabled  IVariant=InternalParameters  DVariant=InternalParameters  IntegratorVariant=Discrete  SatVariant=Enabled  AWVariant=BackCalculation  PCopyVariant=Disabled  TRVariant=Disabled  FdbkBlocksVariant=Forward  IdealPFdbkVariant=Disabled  SatFdbkVariant=Disabled  DerivativeFilterVariant=Differentiator  NVariant=Passthrough  NCopyVariant=Disabled_SignalSpec  FilterICVariant=InternalICsDifferentiator  IntegratorICVariant=InternalICs  ExternalResetVariant=ExternalReset  TRSumVariant=Passthrough  SumFdbkVariant=Disabled  SumVariant=Sum_PID  TsampFilterVariant=InternalTs  TsampNgainVariant=Passthrough  TsampIntegralVariant=Passthrough
  Relational Operator : RelationalOperator  Operator=~=  OutDataTypeStr=boolean  RndMeth=Simplest
  Saturation : Saturate  UpperLimit=10  LowerLimit=-10
  Scope : Scope
  Selector : Selector  InputPortWidth=3  IndexOptions=Index vector (dialog)  Indices=2  OutputSizes=1
  Selector1 : Selector  InputPortWidth=3  IndexOptions=Index vector (dialog)  Indices=3  OutputSizes=1
  Unit Delay : UnitDelay  SampleTime=-1  HasFrameUpgradeWarning=on
  pitch control : Scope  NumInputPorts=5
  trim angle : Constant  Value=2*pi/180
  pitchControl : Outport
  wires:
  FlightParam/1 -> Bus Selector1/1, Bus Selector3/1
  TaskInfo/1 -> Bus Selector5/1
  PID Controller2/1 -> Display1/1, pitch control/3, Divide1/2
  Bus Selector5/3 -> pitch control/1, Add/1  "<heightCmd>"
  Selector/1 -> ?
  Bus Selector3/1 -> Selector/1  "<curEuler>"
  Bus Selector1/1 -> Selector1/1  "<curLLA>"
  Selector1/1 -> pitch control/2, Add/2  "height"
  Bus Selector5/2 -> Compare To Constant/1  "<uavMode>"
  Compare To Constant/1 -> pitch control/5, Divide1/1
  Add/1 -> Saturation/1
  Bus Selector5/1 -> Data Type Conversion2/1  "<flightTaskMode>"
  Relational Operator/1 -> PID Controller2/2, Scope/1
  Data Type Conversion2/1 -> Relational Operator/1, Unit Delay/1
  Unit Delay/1 -> Relational Operator/2
  Saturation/1 -> PID Controller2/1, Display/1, pitch control/4
  Divide1/1 -> Add1/2
  trim angle/1 -> Add1/1
  Add1/1 -> pitchControl/1

== system RefModel_SimpleUavMotion/Subsystem/Pitch Dynamics And InnerLoop ==
  Control : Inport
  1/(2s+1) : discretizing/Discretized Transfer Fcn  Numerator=[1]  Denominator=[0.5 1]  AbsTol=auto  SampleTime=Ts_SimpleUavMotion.Ts_base  method=zoh  Wc=1
      settings: SourceProductBaseCode=SL
  Bus Selector : BusSelector  OutputSignals=pitchControl
  Pitch : Outport
  wires:
  Bus Selector/1 -> 1/(2s+1)/1  "<pitchControl>"
  Control/1 -> Bus Selector/1
  1/(2s+1)/1 -> Pitch/1

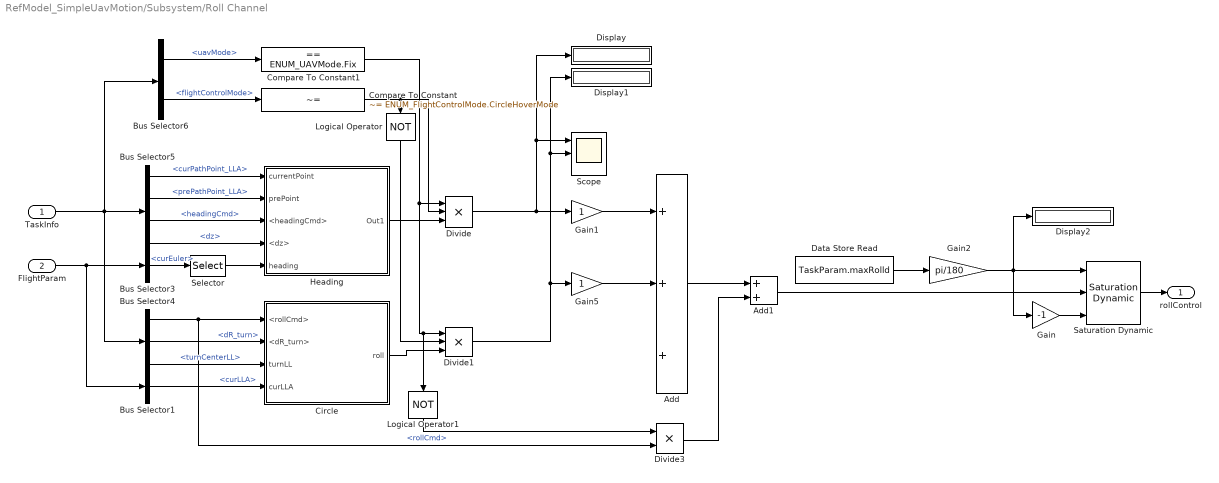
== system RefModel_SimpleUavMotion/Subsystem/Roll Channel ==
  TaskInfo : Inport
  FlightParam : Inport  Port=2
  Add : Sum  Inputs=+++
  Add1 : Sum
  Bus Selector1 : BusSelector  OutputSignals=curLLA
  Bus Selector3 : BusSelector  OutputSignals=curEuler
  Bus Selector4 : BusSelector  OutputSignals=rollCmd,dR_turn,turnCenterLL
  Bus Selector5 : BusSelector  OutputSignals=curPathPoint_LLA,prePathPoint_LLA,headingCmd,dz
  Bus Selector6 : BusSelector  OutputSignals=uavMode,flightControlMode
  Circle : Subsystem
  Compare To Constant : simulink/Logic and Bit Operations/Compare To Constant  relop=~=  const=ENUM_FlightControlMode.CircleHoverMode  OutDataTypeStr=boolean
  Compare To Constant1 : simulink/Logic and Bit Operations/Compare To Constant  relop===  const=ENUM_UAVMode.Fix  OutDataTypeStr=boolean
  Data Store Read : DataStoreRead  DataStoreName=TaskParam  DataStoreElements=TaskParam.maxRolld
  Display : Display
  Display1 : Display
  Display2 : Display
  Divide : Product  Inputs=***
  Divide1 : Product  Inputs=***
  Divide3 : Product  Inputs=**
  Gain : Gain  Gain=-1
  Gain1 : Gain
  Gain2 : Gain  Gain=pi/180
  Gain5 : Gain
  Heading : Subsystem
  Logical Operator : Logic  Operator=NOT  AllPortsSameDT=off  OutDataTypeStr=boolean
  Logical Operator1 : Logic  Operator=NOT  AllPortsSameDT=off  OutDataTypeStr=boolean
  Saturation Dynamic : simulink/Discontinuities/Saturation Dynamic  OutMin=[]  OutMax=[]  OutDataTypeStr=Inherit: Same as second input  OutDataType=fixdt(1, 16)  OutScaling=2^-10  DoSatur=off
  Scope : Scope  NumInputPorts=3
  Selector : Selector  InputPortWidth=3  IndexOptions=Index vector (dialog)  Indices=1  OutputSizes=1
  rollControl : Outport
  wires:
  Add/1 -> Add1/1
  Gain5/1 -> Add/2
  Bus Selector4/2 -> Circle/2(<dR_turn>)  "<dR_turn>"
  Heading/1(Out1) -> Divide/3
  Bus Selector5/3 -> Heading/3(<headingCmd>)  "<headingCmd>"
  Bus Selector4/1 -> Divide3/2, Circle/1(<rollCmd>)  "<rollCmd>"
  Circle/1(roll) -> Divide1/3
  Gain1/1 -> Add/1
  Bus Selector6/2 -> Compare To Constant/1  "<flightControlMode>"
  Logical Operator/1 -> Divide1/2
  Compare To Constant/1 -> Logical Operator/1, Divide/2
  Divide/1 -> Gain1/1, Display/1, Scope/1
  Divide1/1 -> Gain5/1, Display1/1, Scope/2
  TaskInfo/1 -> Bus Selector6/1, Bus Selector5/1, Bus Selector4/1
  FlightParam/1 -> Bus Selector1/1, Bus Selector3/1
  Bus Selector6/1 -> Compare To Constant1/1  "<uavMode>"
  Compare To Constant1/1 -> Divide1/1, Logical Operator1/1, Divide/1
  Selector/1 -> Heading/5(heading)
  Bus Selector3/1 -> Selector/1  "<curEuler>"
  Saturation Dynamic/1 -> rollControl/1
  Logical Operator1/1 -> Divide3/1
  Divide3/1 -> Add1/2
  Add1/1 -> Saturation Dynamic/2
  Bus Selector5/2 -> Heading/2(prePoint)  "<prePathPoint_LLA>"
  Bus Selector5/1 -> Heading/1(currentPoint)  "<curPathPoint_LLA>"
  Bus Selector5/4 -> Heading/4(<dz>)  "<dz>"
  Bus Selector1/1 -> Circle/4(curLLA)  "<curLLA>"
  Bus Selector4/3 -> Circle/3(turnLL)  "<turnCenterLL>"
  Data Store Read/1 -> Gain2/1
  Gain/1 -> Saturation Dynamic/3
  Gain2/1 -> Display2/1, Saturation Dynamic/1, Gain/1

== system RefModel_SimpleUavMotion/Subsystem/Roll Dynamics And InnerLoop ==
  Control : Inport
  1/(2s+1) : discretizing/Discretized Transfer Fcn  Numerator=[1]  Denominator=[0.5 1]  AbsTol=auto  SampleTime=Ts_SimpleUavMotion.Ts_base  method=zoh  Wc=1
      settings: SourceProductBaseCode=SL
  Bus Selector : BusSelector  OutputSignals=rollControl
  MATLAB Function : MATLAB Function  TreatAsAtomicUnit=on
  Roll : Outport
  wires:
  1/(2s+1)/1 -> MATLAB Function/2(y), Roll/1
  Control/1 -> Bus Selector/1
  Bus Selector/1 -> MATLAB Function/1(u), 1/(2s+1)/1  "<rollControl>"

== system RefModel_SimpleUavMotion/Subsystem/Rotor Height Channel ==
  TaskInfo : Inport
  FlightParam : Inport  Port=2
  Bus Selector1 : BusSelector  OutputSignals=curLLA
  Bus Selector3 : BusSelector  OutputSignals=heightCmd,uavMode
  Height Controller : Subsystem
  Selector : Selector  InputPortWidth=3  IndexOptions=Index vector (dialog)  Indices=3  OutputSizes=1
  heightControl : Outport
  wires:
  Bus Selector1/1 -> Selector/1  "<curLLA>"
  Selector/1 -> Height Controller/3(height)
  FlightParam/1 -> Bus Selector1/1
  Bus Selector3/1 -> Height Controller/1(heightCmd)  "<heightCmd>"
  Bus Selector3/2 -> Height Controller/2(uavMode)  "<uavMode>"
  Height Controller/1(heightControl) -> heightControl/1
  TaskInfo/1 -> Bus Selector3/1

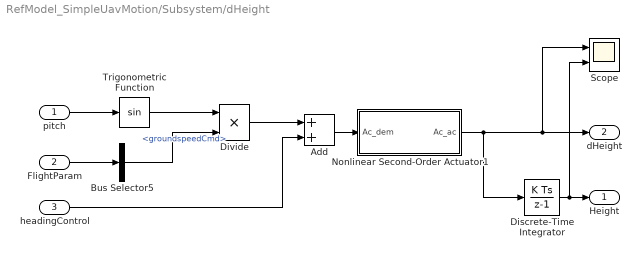
== system RefModel_SimpleUavMotion/Subsystem/dHeight ==
  pitch : Inport
  FlightParam : Inport  Port=2
  headingControl : Inport  Port=3
  Add : Sum
  Bus Selector5 : BusSelector  OutputSignals=groundspeedCmd
  Discrete-Time Integrator : DiscreteIntegrator  SampleTime=-1  ICPrevOutput=DiscIntNeverNeededParam  ICPrevScaledInput=DiscIntNeverNeededParam
  Divide : Product  Inputs=**
  Nonlinear Second-Order Actuator1 : Subsystem  AncestorBlock=aerolibactuator/Nonlinear Second-Order Actuator  mask(NonlinearSecondOrderActuator){wn_fin=1, z_fin=0.7, fin_max=30, fin_min=-30, fin_maxrate=2, fin_act_0=0, fin_act_vel=0}
      mask prompts: wn_fin "aeroblks:aeroblkactuator:blockNonlinearSecondOrderActuatorParamNaturalfrequency"; z_fin "aeroblks:aeroblkactuator:blockNonlinearSecondOrderActuatorParamDampingratio"; fin_max "aeroblks:aeroblkactuator:blockNonlinearSecondOrderActuatorParamMaximumdeflection"; fin_min "aeroblks:aeroblkactuator:blockNonlinearSecondOrderActuatorParamMinimumdeflection"; fin_maxrate "aeroblks:aeroblkactuator:blockNonlinearSecondOrderActuatorParamRatelimit"; fin_act_0 "aeroblks:aeroblkactuator:blockNonlinearSecondOrderActuatorParamInitialposition"; fin_act_vel "aeroblks:aeroblkactuator:blockNonlinearSecondOrderActuatorParamInitialvelocity"
      mask help: aeroblks:aeroblkactuator:blockNonlinearSecondOrderActuatorDesc
      mask init:
      | par = [fin_max fin_min fin_act_0 fin_act_vel fin_maxrate];
      | aeroicon('aeroblkactuator',par)
      mask Help: eval('asbhelp');
      mask Display:
      | port_label('input',1,'A_{demand}','texmode','on');
      | port_label('output',1,'A_{actual}','texmode','on');
  Scope : Scope  NumInputPorts=2
  Trigonometric Function : Trigonometry
  Height : Outport
  dHeight : Outport  Port=2
  wires:
  Add/1 -> Nonlinear Second-Order Actuator1/1(Ac_dem)
  pitch/1 -> Trigonometric Function/1
  Discrete-Time Integrator/1 -> Scope/2, Height/1
  FlightParam/1 -> Bus Selector5/1
  Bus Selector5/1 -> Divide/2  "<groundspeedCmd>"
  Trigonometric Function/1 -> Divide/1
  headingControl/1 -> Add/2
  Divide/1 -> Add/1
  Nonlinear Second-Order Actuator1/1(Ac_ac) -> Discrete-Time Integrator/1, Scope/1, dHeight/1

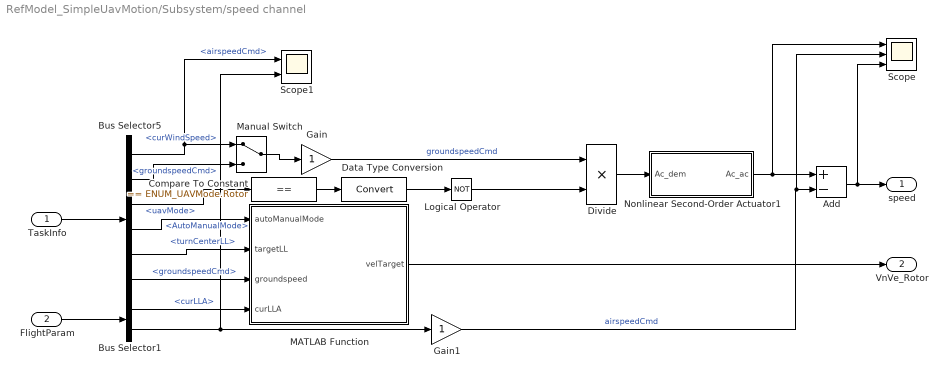
== system RefModel_SimpleUavMotion/Subsystem/speed channel ==
  TaskInfo : Inport
  FlightParam : Inport  Port=2
  Add : Sum  Inputs=+-
  Bus Selector1 : BusSelector  OutputSignals=curLLA,curWindSpeed
  Bus Selector5 : BusSelector  OutputSignals=airspeedCmd,groundspeedCmd,uavMode,AutoManualMode,turnCenterLL,groundspeedCmd
  Compare To Constant : simulink/Logic and Bit Operations/Compare To Constant  relop===  const=ENUM_UAVMode.Rotor  OutDataTypeStr=boolean
  Data Type Conversion : DataTypeConversion
  Divide : Product  Inputs=**
  Gain : Gain
  Gain1 : Gain
  Logical Operator : Logic  Operator=NOT  AllPortsSameDT=off  OutDataTypeStr=boolean
  MATLAB Function : MATLAB Function  TreatAsAtomicUnit=on
  Manual Switch : ManualSwitch
  Nonlinear Second-Order Actuator1 : Subsystem  AncestorBlock=aerolibactuator/Nonlinear Second-Order Actuator  mask(NonlinearSecondOrderActuator){wn_fin=1, z_fin=0.7, fin_max=30, fin_min=0, fin_maxrate=2, fin_act_0=0, fin_act_vel=0}
      mask prompts: wn_fin "aeroblks:aeroblkactuator:blockNonlinearSecondOrderActuatorParamNaturalfrequency"; z_fin "aeroblks:aeroblkactuator:blockNonlinearSecondOrderActuatorParamDampingratio"; fin_max "aeroblks:aeroblkactuator:blockNonlinearSecondOrderActuatorParamMaximumdeflection"; fin_min "aeroblks:aeroblkactuator:blockNonlinearSecondOrderActuatorParamMinimumdeflection"; fin_maxrate "aeroblks:aeroblkactuator:blockNonlinearSecondOrderActuatorParamRatelimit"; fin_act_0 "aeroblks:aeroblkactuator:blockNonlinearSecondOrderActuatorParamInitialposition"; fin_act_vel "aeroblks:aeroblkactuator:blockNonlinearSecondOrderActuatorParamInitialvelocity"
      mask help: aeroblks:aeroblkactuator:blockNonlinearSecondOrderActuatorDesc
      mask init:
      | par = [fin_max fin_min fin_act_0 fin_act_vel fin_maxrate];
      | aeroicon('aeroblkactuator',par)
      mask Help: eval('asbhelp');
      mask Display:
      | port_label('input',1,'A_{demand}','texmode','on');
      | port_label('output',1,'A_{actual}','texmode','on');
  Scope : Scope  NumInputPorts=3
  Scope1 : Scope  NumInputPorts=2
  speed : Outport
  VnVe_Rotor : Outport  Port=2
  wires:
  TaskInfo/1 -> Bus Selector5/1
  Nonlinear Second-Order Actuator1/1(Ac_ac) -> Scope/1, Add/1
  Bus Selector5/3 -> Compare To Constant/1  "<uavMode>"
  FlightParam/1 -> Bus Selector1/1
  Bus Selector5/5 -> MATLAB Function/2(targetLL)  "<turnCenterLL>"
  Compare To Constant/1 -> Data Type Conversion/1
  Bus Selector1/1 -> MATLAB Function/4(curLLA)  "<curLLA>"
  Data Type Conversion/1 -> Logical Operator/1
  Logical Operator/1 -> Divide/2
  Divide/1 -> Nonlinear Second-Order Actuator1/1(Ac_dem)
  MATLAB Function/1(velTarget) -> VnVe_Rotor/1
  Bus Selector5/4 -> MATLAB Function/1(autoManualMode)  "<AutoManualMode>"
  Bus Selector5/6 -> MATLAB Function/3(groundspeed)  "<groundspeedCmd>"
  Gain/1 -> Divide/1  "groundspeedCmd"
  Bus Selector1/2 -> Scope1/2, Gain1/1  "<curWindSpeed>"
  Add/1 -> Scope/3, speed/1
  Gain1/1 -> Scope/2, Add/2  "airspeedCmd"
  Bus Selector5/1 -> Manual Switch/1, Scope1/1  "<airspeedCmd>"
  Manual Switch/1 -> Gain/1
  Bus Selector5/2 -> Manual Switch/2  "<groundspeedCmd>"

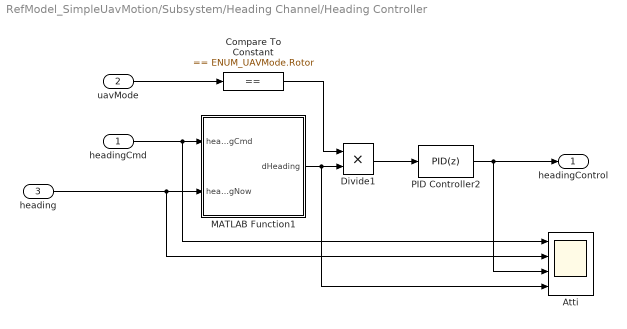
== system RefModel_SimpleUavMotion/Subsystem/Heading Channel/Heading Controller ==
  headingCmd : Inport
  uavMode : Inport  Port=2
  heading : Inport  Port=3
  Atti : Scope  NumInputPorts=4
  Compare To Constant : simulink/Logic and Bit Operations/Compare To Constant  relop===  const=ENUM_UAVMode.Rotor  OutDataTypeStr=boolean
  Divide1 : Product  Inputs=**
  MATLAB Function1 : MATLAB Function  TreatAsAtomicUnit=on
  PID Controller2 : simulink/Continuous/PID Controller  Controller=PID  Form=Parallel  TimeDomain=Discrete-time  UseExternalTs=off  SampleTime=Ts_SimpleUavMotion.Ts_base  IntegratorMethod=Forward Euler  FilterMethod=Forward Euler  ControllerParametersSource=internal  P=1e-3  I=0  D=0  UseFilter=on  N=50  TunerSelectOption=Transfer Function Based (PID Tuner App)  InitialConditionSource=internal  InitialConditionForIntegrator=0  InitialConditionForFilter=0  DifferentiatorICPrevScaledInput=0  ExternalReset=none  TrackingMode=off  Kt=1  LimitOutput=off  UpperSaturationLimit=50*pi/180  LowerSaturationLimit=-50*pi/180  LinearizeAsGain=on  AntiWindupMode=none  Kb=1  POutMin=[]  POutMax=[]  IOutMin=[]  IOutMax=[]  DOutMin=[]  DOutMax=[]  NOutMin=[]  NOutMax=[]  SumOutMin=[]  SumOutMax=[]  SaturationOutMin=[]  SaturationOutMax=[]  PParamMin=[]  PParamMax=[]  IParamMin=[]  IParamMax=[]  DParamMin=[]  DParamMax=[]  NParamMin=[]  NParamMax=[]  KbParamMin=[]  KbParamMax=[]  KtParamMin=[]  KtParamMax=[]  KbOutMin=[]  KbOutMax=[]  KtOutMin=[]  KtOutMax=[]  IntegratorOutMin=[]  IntegratorOutMax=[]  FilterOutMin=[]  FilterOutMax=[]  SumI1OutMin=[]  SumI1OutMax=[]  SumI2OutMin=[]  SumI2OutMax=[]  SumI3OutMin=[]  SumI3OutMax=[]  SumI4OutMin=[]  SumI4OutMax=[]  SumDOutMin=[]  SumDOutMax=[]  DifferentiatorOutMin=[]  DifferentiatorOutMax=[]  FilterDiffOutCoefMin=[]  FilterDiffOutCoefMax=[]  ReciprocalOutMin=[]  ReciprocalOutMax=[]  SumDenOutMin=[]  SumDenOutMax=[]  SumNumOutMin=[]  SumNumOutMax=[]  DivideOutMin=[]  DivideOutMax=[]  UdiffTsProdOutMin=[]  UdiffTsProdOutMax=[]  NTsProdOutMin=[]  NTsProdOutMax=[]  UintegralTsProdOutMin=[]  UintegralTsProdOutMax=[]  UngainTsProdOutMin=[]  UngainTsProdOutMax=[]  IntegratorContinuousStateAttributes=''  IntegratorStateMustResolveToSignalObject=off  IntegratorRTWStateStorageClass=Auto  FilterContinuousStateAttributes=''  FilterStateMustResolveToSignalObject=off  FilterRTWStateStorageClass=Auto  ParallelPVariant=InternalParameters  IdealPVariant=Disabled  IVariant=InternalParameters  DVariant=InternalParameters  IntegratorVariant=Discrete  SatVariant=Disabled  AWVariant=Passthrough  PCopyVariant=Disabled  TRVariant=Disabled  FdbkBlocksVariant=Forward  IdealPFdbkVariant=Disabled  SatFdbkVariant=Disabled  DerivativeFilterVariant=ForwardEulerFilter  NVariant=InternalParameters  NCopyVariant=Disabled  FilterICVariant=InternalICsFilter  IntegratorICVariant=InternalICs  ExternalResetVariant=Disabled  TRSumVariant=Passthrough  SumFdbkVariant=Disabled  SumVariant=Sum_PID  TsampFilterVariant=InternalTs  TsampNgainVariant=Passthrough  TsampIntegralVariant=Passthrough
  headingControl : Outport
  wires:
  headingCmd/1 -> MATLAB Function1/1(headingCmd), Atti/1
  uavMode/1 -> Compare To Constant/1
  Compare To Constant/1 -> Divide1/1
  PID Controller2/1 -> headingControl/1, Atti/3
  heading/1 -> MATLAB Function1/2(headingNow), Atti/2
  Divide1/1 -> PID Controller2/1
  MATLAB Function1/1(dHeading) -> Atti/4, Divide1/2

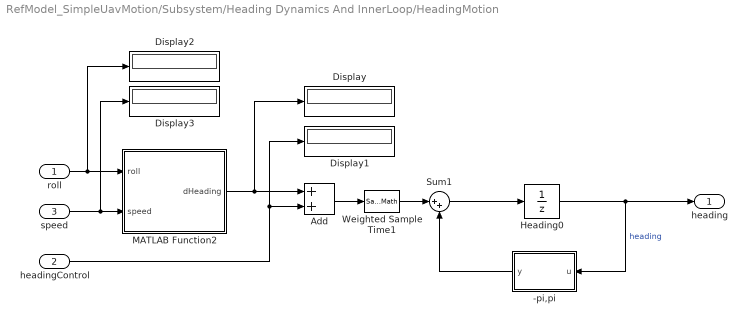
== system RefModel_SimpleUavMotion/Subsystem/Heading Dynamics And InnerLoop/HeadingMotion ==
  roll : Inport
  headingControl : Inport  Port=2
  speed : Inport  Port=3
  -pi,pi : MATLAB Function  TreatAsAtomicUnit=on
  Add : Sum
  Display{,1..3} (4 alike) : Display
  Heading0 : UnitDelay  SampleTime=-1  HasFrameUpgradeWarning=on
  MATLAB Function2 : MATLAB Function  TreatAsAtomicUnit=on
  Sum1 : Sum  Inputs=|++
  Weighted Sample Time1 : SampleTimeMath  TsampMathOp=*
  heading : Outport
  wires:
  Sum1/1 -> Heading0/1
  roll/1 -> Display2/1, MATLAB Function2/1(roll)
  Heading0/1 -> heading/1, -pi,pi/1(u)  "heading"
  speed/1 -> Display3/1, MATLAB Function2/2(speed)
  MATLAB Function2/1(dHeading) -> Display/1, Add/1
  Add/1 -> Weighted Sample Time1/1
  headingControl/1 -> Display1/1, Add/2
  Weighted Sample Time1/1 -> Sum1/1
  -pi,pi/1(y) -> Sum1/2

== system RefModel_SimpleUavMotion/Subsystem/Roll Channel/Circle ==
  <rollCmd> : Inport
  <dR_turn> : Inport  Port=2
  turnLL : Inport  Port=3
  curLLA : Inport  Port=4
  Add1 : Sum
  Gain4 : Gain  Gain=-1
  PID Controller1 : simulink/Continuous/PID Controller  Controller=PID  Form=Parallel  TimeDomain=Discrete-time  UseExternalTs=off  SampleTime=Ts_SimpleUavMotion.Ts_base  IntegratorMethod=Forward Euler  FilterMethod=Forward Euler  ControllerParametersSource=internal  P=0.05  I=0  D=0.25  UseFilter=on  N=24.542109027781645  TunerSelectOption=Transfer Function Based (PID Tuner App)  ZeroCross=off  InitialConditionSource=internal  InitialConditionForIntegrator=0  InitialConditionForFilter=0  DifferentiatorICPrevScaledInput=0  ExternalReset=none  TrackingMode=off  Kt=1  LimitOutput=off  UpperSaturationLimit=0.5  LowerSaturationLimit=-0.5  LinearizeAsGain=on  AntiWindupMode=none  Kb=1  POutMin=[]  POutMax=[]  IOutMin=[]  IOutMax=[]  DOutMin=[]  DOutMax=[]  NOutMin=[]  NOutMax=[]  SumOutMin=[]  SumOutMax=[]  SaturationOutMin=[]  SaturationOutMax=[]  PParamMin=[]  PParamMax=[]  IParamMin=[]  IParamMax=[]  DParamMin=[]  DParamMax=[]  NParamMin=[]  NParamMax=[]  KbParamMin=[]  KbParamMax=[]  KtParamMin=[]  KtParamMax=[]  KbOutMin=[]  KbOutMax=[]  KtOutMin=[]  KtOutMax=[]  IntegratorOutMin=[]  IntegratorOutMax=[]  FilterOutMin=[]  FilterOutMax=[]  SumI1OutMin=[]  SumI1OutMax=[]  SumI2OutMin=[]  SumI2OutMax=[]  SumI3OutMin=[]  SumI3OutMax=[]  SumI4OutMin=[]  SumI4OutMax=[]  SumDOutMin=[]  SumDOutMax=[]  DifferentiatorOutMin=[]  DifferentiatorOutMax=[]  FilterDiffOutCoefMin=[]  FilterDiffOutCoefMax=[]  ReciprocalOutMin=[]  ReciprocalOutMax=[]  SumDenOutMin=[]  SumDenOutMax=[]  SumNumOutMin=[]  SumNumOutMax=[]  DivideOutMin=[]  DivideOutMax=[]  UdiffTsProdOutMin=[]  UdiffTsProdOutMax=[]  NTsProdOutMin=[]  NTsProdOutMax=[]  UintegralTsProdOutMin=[]  UintegralTsProdOutMax=[]  UngainTsProdOutMin=[]  UngainTsProdOutMax=[]  IntegratorContinuousStateAttributes=''  IntegratorStateMustResolveToSignalObject=off  IntegratorRTWStateStorageClass=Auto  FilterContinuousStateAttributes=''  FilterStateMustResolveToSignalObject=off  FilterRTWStateStorageClass=Auto  ParallelPVariant=InternalParameters  IdealPVariant=Disabled  IVariant=InternalParameters  DVariant=InternalParameters  IntegratorVariant=Discrete  SatVariant=Disabled  AWVariant=Passthrough  PCopyVariant=Disabled  TRVariant=Disabled  FdbkBlocksVariant=Forward  IdealPFdbkVariant=Disabled  SatFdbkVariant=Disabled  DerivativeFilterVariant=ForwardEulerFilter  NVariant=InternalParameters  NCopyVariant=Disabled  FilterICVariant=InternalICsFilter  IntegratorICVariant=InternalICs  ExternalResetVariant=Disabled  TRSumVariant=Passthrough  SumFdbkVariant=Disabled  SumVariant=Sum_PID  TsampFilterVariant=InternalTs  TsampNgainVariant=Passthrough  TsampIntegralVariant=Passthrough
  roll : Outport
  wires:
  <dR_turn>/1 -> Gain4/1
  Add1/1 -> roll/1  "roll"
  PID Controller1/1 -> Add1/2
  <rollCmd>/1 -> Add1/1
  Gain4/1 -> PID Controller1/1
